simulink model "Rear"  (Simulink 8.1)
settings: Solver=ode45  StartTime=0.0  StopTime=10.0  RelTol=1e-3
settings Model: Creator=Brian  LastModifiedBy=Brian
settings DataIOCC: SignalLoggingSaveFormat=Dataset
settings OptimizationCC: ExpressionDepthLimit=128
settings DebuggingCC: FcnCallInpInsideContextMsg=EnableAllAsError
settings GRTTargetCC: CombineOutputUpdateFcns=on  GRTInterface=off

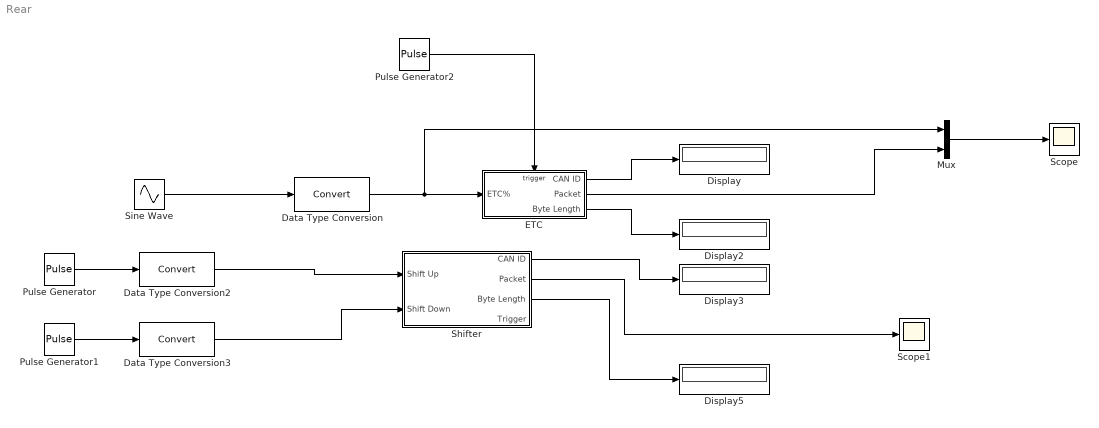
== system Rear ==
  Data Type Conversion : DataTypeConversion
  Data Type Conversion2 : DataTypeConversion
  Data Type Conversion3 : DataTypeConversion
  Display{,2..3,5} (4 alike) : Display
      settings: Format=hex (Stored Integer)
  ETC : Subsystem
  Mux : Mux  Inputs=2
  Pulse Generator : DiscretePulseGenerator  PulseType=Time based  PulseWidth=5  PhaseDelay=.5
  Pulse Generator1 : DiscretePulseGenerator  PulseType=Time based  PulseWidth=5
  Pulse Generator2 : DiscretePulseGenerator  PulseType=Time based  Period=.05  PulseWidth=5
  Scope : Scope
  Scope1 : Scope
  Shifter : Subsystem
  Sine Wave : Sin  Amplitude=45  Bias=45  Frequency=3.14  SampleTime=0
  wires:
  ETC/1(CAN ID) -> Display/1
  ETC/2(Packet) -> Mux/2
  ETC/3(Byte Length) -> Display2/1
  Shifter/1(CAN ID) -> Display3/1
  Shifter/3(Byte Length) -> Display5/1
  Sine Wave/1 -> Data Type Conversion/1
  Pulse Generator/1 -> Data Type Conversion2/1
  Pulse Generator1/1 -> Data Type Conversion3/1
  Data Type Conversion/1 -> Mux/1, ETC/1(ETC%)
  Mux/1 -> Scope/1
  Data Type Conversion2/1 -> Shifter/1(Shift Up)
  Data Type Conversion3/1 -> Shifter/2(Shift Down)
  Shifter/2(Packet) -> Scope1/1
  Pulse Generator2/1 -> ETC/Trigger

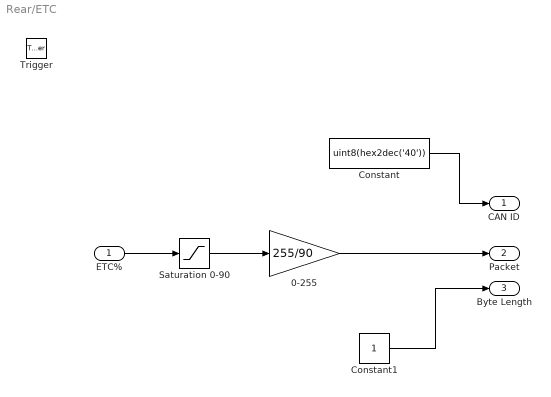
== system Rear/ETC ==
  ETC% : Inport  OutDataTypeStr=uint8
  Trigger : TriggerPort  PortDimensions=1
  0-255 : Gain  Gain=255/90  OutDataTypeStr=uint8
  Constant : Constant  Value=uint8(hex2dec('40'))  OutDataTypeStr=uint8
  Constant1 : Constant  OutDataTypeStr=uint8
  Saturation 0-90 : Saturate  UpperLimit=90  LowerLimit=0
  CAN ID : Outport
  Packet : Outport  Port=2
  Byte Length : Outport  Port=3
  wires:
  Constant/1 -> CAN ID/1
  ETC%/1 -> Saturation 0-90/1
  Saturation 0-90/1 -> 0-255/1
  0-255/1 -> Packet/1
  Constant1/1 -> Byte Length/1

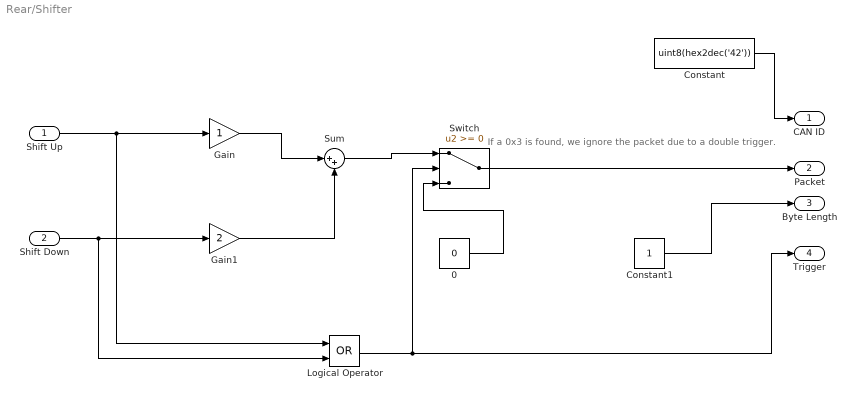
== system Rear/Shifter ==
  note: If a 0x3 is found, we ignore the packet due to a double trigger.
  Shift Up : Inport  OutDataTypeStr=boolean
  Shift Down : Inport  Port=2  OutDataTypeStr=boolean
  0 : Constant  Value=0  OutDataTypeStr=uint8
  Constant : Constant  Value=uint8(hex2dec('42'))  OutDataTypeStr=uint8
  Constant1 : Constant  OutDataTypeStr=uint8
  Gain : Gain  OutDataTypeStr=uint8
  Gain1 : Gain  Gain=2  OutDataTypeStr=uint8
  Logical Operator : Logic  Operator=OR  AllPortsSameDT=off  OutDataTypeStr=boolean
  Sum : Sum  Inputs=|++
  Switch : Switch
  CAN ID : Outport
  Packet : Outport  Port=2  OutDataTypeStr=uint8
  Byte Length : Outport  Port=3
  Trigger : Outport  Port=4
  wires:
  Constant/1 -> CAN ID/1
  Constant1/1 -> Byte Length/1
  Shift Up/1 -> Gain/1, Logical Operator/1
  Shift Down/1 -> Gain1/1, Logical Operator/2
  Logical Operator/1 -> Switch/2, Trigger/1
  Switch/1 -> Packet/1
  0/1 -> Switch/3
  Gain1/1 -> Sum/2
  Gain/1 -> Sum/1
  Sum/1 -> Switch/1
